simulink model "TwoToOneMultiplexor"  (R2017b)
settings: Solver=VariableStepAuto  StartTime=0.0  StopTime=10.0  RelTol=1e-3
settings Model: Creator=Ray  LastModifiedBy=Ray

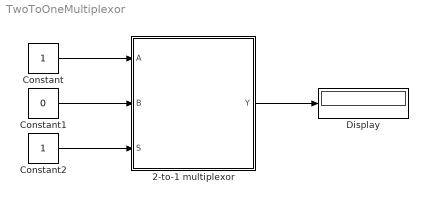
== system TwoToOneMultiplexor ==
  2-to-1 multiplexor : Subsystem
  Constant : Constant  OutDataTypeStr=boolean  SampleTime=1
  Constant1 : Constant  Value=0  OutDataTypeStr=boolean  SampleTime=1
  Constant2 : Constant  OutDataTypeStr=boolean  SampleTime=1
  Display : Display
  wires:
  Constant/1 -> 2-to-1 multiplexor/1(A)
  Constant1/1 -> 2-to-1 multiplexor/2(B)
  Constant2/1 -> 2-to-1 multiplexor/3(S)
  2-to-1 multiplexor/1(Y) -> Display/1

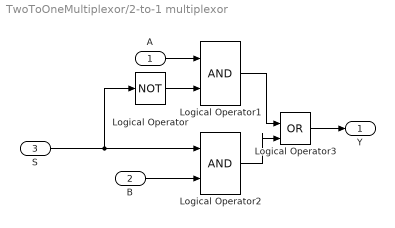
== system TwoToOneMultiplexor/2-to-1 multiplexor ==
  A : Inport  OutDataTypeStr=boolean  SampleTime=1
  B : Inport  Port=2  OutDataTypeStr=boolean  SampleTime=1
  S : Inport  Port=3  OutDataTypeStr=boolean  SampleTime=1
  Logical Operator : Logic  Operator=NOT  IconShape=distinctive  AllPortsSameDT=off  OutDataTypeStr=boolean
  Logical Operator1 : Logic  IconShape=distinctive  AllPortsSameDT=off  OutDataTypeStr=boolean
  Logical Operator2 : Logic  IconShape=distinctive  AllPortsSameDT=off  OutDataTypeStr=boolean
  Logical Operator3 : Logic  Operator=OR  IconShape=distinctive  AllPortsSameDT=off  OutDataTypeStr=boolean
  Y : Outport
  wires:
  Logical Operator2/1 -> Logical Operator3/2
  Logical Operator1/1 -> Logical Operator3/1
  Logical Operator3/1 -> Y/1
  A/1 -> Logical Operator1/1
  S/1 -> Logical Operator2/1, Logical Operator/1
  B/1 -> Logical Operator2/2
  Logical Operator/1 -> Logical Operator1/2
